simulink model "Mesh"  (Simulink 7.9)
settings: Solver=ode4  StartTime=0.0  StopTime=0.5  FixedStep=0.0001  RelTol=1e-10
values from neighbouring files (symbols this model uses):
  b = 0.01    [Initialization.m]
  deltap = -0.003    [Initialization.m]
  Fs = 70    [Initialization.m]
  I0 = 0    [Initialization.m]
  ig2 = 3.704    [Initialization.m]
  Jg2 = 0.7    [Initialization.m]
  mg2 = 18.1    [Initialization.m]
  ms = 3.2    [Initialization.m]
  px0 = -0.0165    [Initialization.m]
  py0 = 0.003    [Initialization.m]
  Rs = 0.08    [Initialization.m]
  Tf = 1    [Initialization.m]
  theta = pi*(36/180)    (= 0.628318530718)    [Initialization.m]
  vx0 = 0    [Initialization.m]
  vy0 = 0    [Initialization.m]
  zeta = 0.9    [Initialization.m]
libraries: simulink x1
settings Model: Creator=Hongxu Chen  LastModifiedBy=Administrator

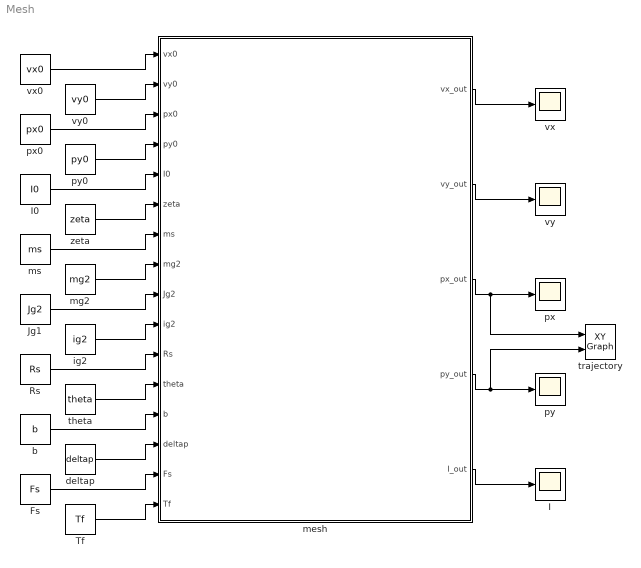
== system Mesh ==
  Fs : Constant  Value=Fs
  I : Scope
      settings: SaveName=ScopeData4
  I0 : Constant  Value=I0
  Jg1 : Constant  Value=Jg2
  Rs : Constant  Value=Rs
  Tf : Constant  Value=Tf
  b : Constant  Value=b
  deltap : Constant  Value=deltap
  ig2 : Constant  Value=ig2
  mesh : Stateflow chart  TreatAsAtomicUnit=on
  mg2 : Constant  Value=mg2
  ms : Constant  Value=ms
  px : Scope
      settings: TimeRange=1  YMin=-2  YMax=12  SaveName=ScopeData2
  px0 : Constant  Value=px0
  py : Scope
      settings: SaveName=ScopeData3
  py0 : Constant  Value=py0
  theta : Constant  Value=theta
  trajectory : simulink/Sinks/XY Graph  xmin=-0.02  xmax=0  ymin=-0.015  ymax=0.015  st=-1
  vx : Scope
  vx0 : Constant  Value=vx0
  vy : Scope
  vy0 : Constant  Value=vy0
  zeta : Constant  Value=zeta
  wires:
  vx0/1 -> mesh/1(vx0)
  vy0/1 -> mesh/2(vy0)
  px0/1 -> mesh/3(px0)
  py0/1 -> mesh/4(py0)
  I0/1 -> mesh/5(I0)
  zeta/1 -> mesh/6(zeta)
  ms/1 -> mesh/7(ms)
  mg2/1 -> mesh/8(mg2)
  Jg1/1 -> mesh/9(Jg2)
  ig2/1 -> mesh/10(ig2)
  Rs/1 -> mesh/11(Rs)
  theta/1 -> mesh/12(theta)
  b/1 -> mesh/13(b)
  deltap/1 -> mesh/14(deltap)
  Fs/1 -> mesh/15(Fs)
  Tf/1 -> mesh/16(Tf)
  mesh/1(vx_out) -> vx/1
  mesh/2(vy_out) -> vy/1
  mesh/3(px_out) -> px/1, trajectory/1
  mesh/4(py_out) -> py/1, trajectory/2
  mesh/5(I_out) -> I/1

== stateflow chart mesh ==
  settings: updateMethod=CONTINUOUS  executeAtInitialization=1  initializeOutput=1
  state move_free
    du:
    vx_dot=Fs/ms;
    vy_dot=-Rs*Tf/Jg2;
    px_dot=vx;
    py_dot=vy;
    I_dot=0;
    vx_out=vx;
    vy_out=vy;
    px_out=px;
    py_out=py;
    I_out=I;
  state meshed
    du:
    vx_dot=0;
    vy_dot=0;
    px_dot=vx;
    py_dot=vy;
    I_dot=0;
    vx_out=vx;
    vy_out=vy;
    px_out=px;
    py_out=py;
    I_out=I;
  (default) -> move_free : {
      | vx=vx0;
      | vy=vy0;
      | px=px0;
      | py=py0;
      | I=I0;}
  move_free -> move_free [order 2] : [py<=px*tan(theta) && vx*sin(theta)-vy*cos(theta)>0]
      | {I=I+(vx*sin(theta)-vy*cos(theta))*(zeta+1)*ms*mg2/(ms*(cos(theta)^2)+mg2*(sin(theta)^2));
      | vx_r=(vx*(ms*cos(theta)^2-mg2*zeta*sin(theta)^2)+vy*((zeta+1)*mg2*sin(theta)*cos(theta)))/(ms*(cos(theta)^2)+mg2*(sin(theta)^2));
      | vy_r=(vx*((zeta+1)*ms*sin(theta)*cos(theta))+vy*(mg2*sin(theta)^2-ms*zeta*cos(theta)^2))/(ms*(cos(theta)^2)+mg2*(sin(theta)^2));
      | vx=vx_r;vy=vy_r;
      | px=px;py=py;
      | }
  move_free -> move_free [order 1] : [py>=-px*tan(theta) && vx*sin(theta)+vy*cos(theta)>0]
      | {I=I+(vx*sin(theta)+vy*cos(theta))*(zeta+1)*ms*mg2/(ms*(cos(theta)^2)+mg2*(sin(theta)^2));
      | vx_r=(vx*(ms*cos(theta)^2-mg2*zeta*sin(theta)^2)+vy*(-(zeta+1)*mg2*sin(theta)*cos(theta)))/(ms*(cos(theta)^2)+mg2*(sin(theta)^2));
      | vy_r=(vx*(-(zeta+1)*ms*sin(theta)*cos(theta))+vy*(mg2*sin(theta)^2-ms*zeta*cos(theta)^2))/(ms*(cos(theta)^2)+mg2*(sin(theta)^2));
      | vx=vx_r;vy=vy_r;
      | px=px;py=py;
      | }
  move_free -> meshed [order 3] : [px>=deltap]
      | {I=I+ms*abs(vx)+ms*abs(vy);
      | vx=0;vy=0;
      | px=px;py=py;
      | }
  data: vx_out output double size=1; vy_out output double size=1; px_out output double size=1; py_out output double size=1; vx local double; vy local double; px local double; py local double; vx0 input double; vy0 input double; px0 input double; py0 input double; I0 input double; zeta input double; ms input double; mg2 input double; Jg2 input double; ig2 input double; Rs input double; theta input double; b input double; deltap input double; Fs input double; Tf input double; I local double size=1 =0; I_out output double size=1; vx_r local double; vy_r local double
  data vx settings: updateMethod=SF_CONTINUOUS_TIME_DATA
  data vy settings: updateMethod=SF_CONTINUOUS_TIME_DATA
  data px settings: updateMethod=SF_CONTINUOUS_TIME_DATA
  data py settings: updateMethod=SF_CONTINUOUS_TIME_DATA
  data I settings: updateMethod=SF_CONTINUOUS_TIME_DATA
  data vx_r settings: updateMethod=SF_CONTINUOUS_TIME_DATA
  data vy_r settings: updateMethod=SF_CONTINUOUS_TIME_DATA
